simulink model "w1prob8"  (R2020a)
settings: Solver=VariableStepAuto  StartTime=0.0  StopTime=10.0  RelTol=1e-3
settings Model: Creator=Anjali123  LastModifiedBy=Anjali123

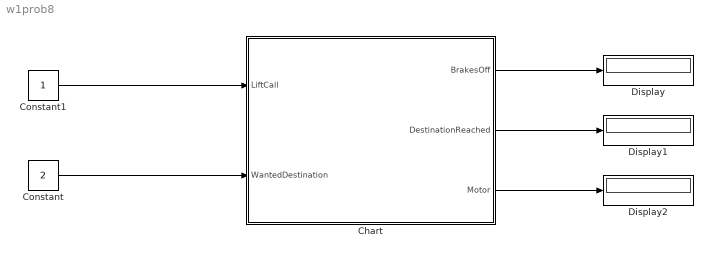
== system w1prob8 ==
  Chart : Stateflow chart  TreatAsAtomicUnit=on
  Constant : Constant  Value=2
  Constant1 : Constant
  Display : Display
  Display1 : Display
  Display2 : Display
  wires:
  Constant1/1 -> Chart/1(LiftCall)
  Constant/1 -> Chart/2(WantedDestination)
  Chart/1(BrakesOff) -> Display/1
  Chart/2(DestinationReached) -> Display1/1
  Chart/3(Motor) -> Display2/1

== stateflow chart w1prob8/Chart ==
  state Stopped
    state Stopped_and_waiting
      state Initialising
        entry: Motor = false; BrakesOff = false; Doors = false;
        CommandConsidered = false;
      state FixingDestination
        LastDestination = WantedDestination;
      state SettingUp
        entry:
        Up = true;
      state SettingDown
        entry:
        Up = false;
      state CommandAccepted
        CommandConsidered = true;
      Initialising -> Initialising [order 2] : [~LiftCall && ~CommandConsidered]
      (default) -> Initialising
      Initialising -> FixingDestination [order 1] : [LiftCall]
      FixingDestination -> SettingUp [order 1] : [CurrentPosition < LastDestination]
      FixingDestination -> SettingDown [order 2] : [CurrentPosition > LastDestination]
      SettingUp -> CommandAccepted
      SettingDown -> CommandAccepted
    state Stopped_at_destination
      state StoppingLift
        entry: Motor = false; BrakesOff = false;
      state ErrorState
        entry:
        Doors = false;
      state OpeningDoors
        entry:
        DestinationReached = CurrentPosition;
        Doors = true;
      (default) -> StoppingLift
      StoppingLift -> OpeningDoors [order 1] : [CurrentPosition == LastDestination]
      StoppingLift -> ErrorState [order 2] : [CurrentPosition ~= LastDestination]
    (default) -> Stopped_and_waiting
    Stopped_at_destination -> Stopped_and_waiting : [Doors]
    FixingDestination -> Stopped_at_destination [order 3] : [CurrentPosition == LastDestination]
  state Moving
    state StartingMotor
      entry: Motor = true; BrakesOff = true; Doors = false;
    state MovingUp
      entry:
      CurrentPosition = CurrentPosition + 1;
    state MovingDown
      entry:
      CurrentPosition = CurrentPosition - 1;
    (default) -> StartingMotor
    StartingMotor -> MovingUp [order 1] : [Up]
    StartingMotor -> MovingDown [order 2] : [~Up]
    MovingUp -> MovingUp : [CurrentPosition < LastDestination]
    MovingDown -> MovingDown : [CurrentPosition > LastDestination]
  (default) -> Stopped : {CurrentPosition = 0;}
  CommandAccepted -> Moving : [CommandConsidered]
  Moving -> Stopped_at_destination : [CurrentPosition == LastDestination]
  data: LiftCall input; WantedDestination input; BrakesOff output; DestinationReached output; Motor output; CommandConsidered local; CurrentPosition local; Doors local; LastDestination local; Up local
